simulink model "ztfk"  (R2021a)
settings: Solver=ode45  StartTime=0.0  StopTime=10.0  RelTol=1e-3  EnableMultiTasking=on
values from neighbouring files (symbols this model uses):
  K = [  -60.6992 -316.1745  -30.0745  -33.7643]    [daolibai.m]    (also in dlfun.m = [ -60.6992 -316.1745  -30.0745  -33.7643]; fang_daolibai.m = place(A,B,P); xiankongdlb.m = place(A,B,P))
settings Model: Creator=secn06  LastModifiedBy=HanDong
settings SolverCC: AlgebraicLoopSolver=TrustRegion
settings DataIOCC: LimitDataPoints=on  SaveFormat=Array  ReturnWorkspaceOutputs=off
settings OptimizationCC: LifeSpan=inf
settings DebuggingCC: SolverPrmCheckMsg=warning  SFUnexpectedBacktrackingDiag=warning  SFNoUnconditionalDefaultTransitionDiag=warning  SFExecutionAtInitializationDiag=none  SFMachineParentedDataDiag=warning  ArithmeticOperatorsInVariantConditions=warning
settings HardwareCC: ProdBitPerPointer=32  ProdBitPerSizeT=32  ProdBitPerPtrDiffT=32  ProdLargestAtomicFloat=None  ProdIntDivRoundTo=Undefined  ProdEndianess=Unspecified  ProdWordSize=32  ProdHWDeviceType=32-bit Generic
settings ModelReferenceCC: PropagateSignalLabelsOutOfModel=off
settings SFSimCC: SimUseLocalCustomCode=off  CustomCodeUndefinedFunction=UseInterfaceOnly
settings RTWCC: RTWUseLocalCustomCode=off
settings CodeAppCC: StateflowObjectComments=on
settings GRTTargetCC: TargetLangStandard=C89/C90 (ANSI)
settings ConfigComp: CovMetricSettings=dw  CovSaveCumulativeToWorkspaceVar=on  CovSaveSingleToWorkspaceVar=on  CovExternalEMLEnable=off  CovSFcnEnable=off

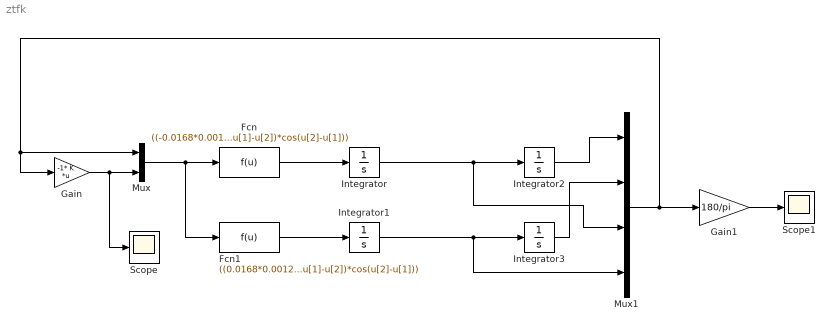
== system ztfk ==
  Fcn : Fcn  Expr=((-0.0168*0.001)*u[3]+(0.001*0.0012*cos(u[2]-u[1]))*u[4]+0.0012*0.0012*sin(u[2]-u[1])* cos(u[2]-u[1])*u[3]*u[3]-0.0012*0.001*sin(u[1]-u[2])*u[4]*u[4]+0.2979*0.001*sin(u[1])-0.0612*0.0012*sin(u[2])*cos(u[2]-u[1])+0.0236*0.001*u[5])/(0.0061*0.001-0.0012*0.0012*cos(u[1]-u[2])*cos(u[2]-u[1]))
  Fcn1 : Fcn  Expr=((0.0168*0.0012*cos(u[1]-u[2]))*u[3]-(0.0061*0.001)*u[4]-0.0061*0.0012*sin(u[2]-u[1])*u[3]*u[3]+0.0012*0.0012*sin(u[1]-u[2])*cos(u[1]-u[2])*u[4]*u[4]-0.2979*0.0012*sin(u[1])*cos(u[1]-u[2])+0.0061*0.0612*sin(u[2])-0.0012*cos(u[1]-u[2])*0.0236*u[5])/(0.0061*0.001-0.0012*0.0012*cos(u[1]-u[2])*cos(u[2]-u[1]))
  Gain : Gain  Gain=-1* K  Multiplication=Matrix(K*u)
  Gain1 : Gain  Gain=180/pi
  Integrator : Integrator
  Integrator1 : Integrator
  Integrator2 : Integrator  InitialCondition=0.01
  Integrator3 : Integrator  InitialCondition=0.01
  Mux : Mux  Inputs=2
  Mux1 : Mux
  Scope : Scope
  Scope1 : Scope
  wires:
  Gain/1 -> Scope/1, Mux/2
  Mux/1 -> Fcn1/1, Fcn/1
  Fcn/1 -> Integrator/1
  Fcn1/1 -> Integrator1/1
  Integrator1/1 -> Integrator3/1, Mux1/4
  Integrator/1 -> Integrator2/1, Mux1/3
  Integrator2/1 -> Mux1/1
  Integrator3/1 -> Mux1/2
  Mux1/1 -> Gain/1, Mux/1, Gain1/1
  Gain1/1 -> Scope1/1
